simulink model "Approach2_ADAS_SimuEnv_Students"  (R2023b)
settings: Solver=FixedStepDiscrete  StartTime=0.0  StopTime=Time(end)  FixedStep=Te  RelTol=1e-3
undefined symbols (not defined in the file): b, DiscIntNeverNeededParam, phieq, phiini, Te, xini, yini
settings Model: Creator=a004139  LastModifiedBy=merte
settings SolverCC: AlgebraicLoopSolver=TrustRegion
settings DataIOCC: SaveOutput=off  SignalLogging=off  DSMLogging=off  SaveTime=off  ReturnWorkspaceOutputs=off  ReturnWorkspaceOutputsName=SimOut
settings DebuggingCC: UnconnectedInputMsg=warning  UnconnectedOutputMsg=warning  UnconnectedLineMsg=warning
settings ModelReferenceCC: EnableRefExpFcnMdlSchedulingChecks=on
settings RTWCC: DLArmComputeVersion=19.05

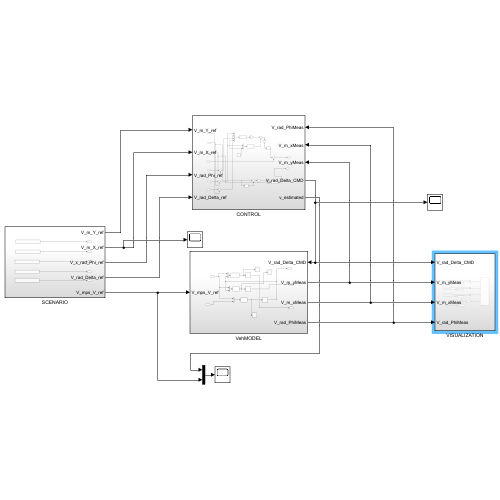
[thumbnail: Simulink's stored preview of the top-level diagram]
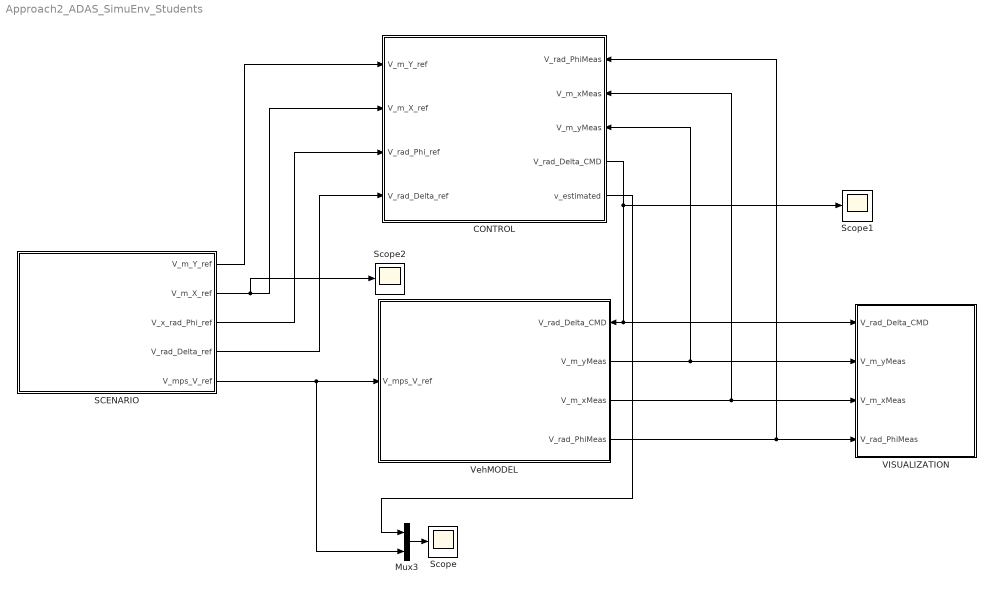
== system Approach2_ADAS_SimuEnv_Students ==
  CONTROL : Subsystem
      settings: PortSchema="{\"entries\":[{\"content\":{\"sides\":[{\"content\":{\"connectorIds\":[\"In1\",\"In2\",\"In3\",\"In4\"]},\"type\":\"ConnectorPlacement.EquallySpacedRectSide\",\"uuid\":\"0f23f3c4-7533-49c9-95fd-578963f4a754\"},{\"content\":{\"connectorIds\":[\"In5\",\"In6\",\"In7\",\"Out1\",\"Out2\"],\"side\":\"RIGHT\"},\"type\":\"ConnectorPlacement.EquallySpacedRectSide\",\"uuid\":\"9ec2fbe1-bc80-46e0-b9ca-3ad9a8a7d04a\"},{\"content\":{\"side\":\"TOP\"},\"type\":\"ConnectorPlacement.EquallySpacedRectSide\",\"uuid\":\"b91c010f-db5d-47ed-ad65-4a9135c33450\"}]},\"type\":\"ConnectorPlacement.EquallySpacedConnector\",\"uuid\":\"9aa72db9-4388-4ef7-aaa1-98aa5bf9b2fd\"}],\"packageUris\":[\"http://schema.mathworks.com/mf0/Connector/R2020b\"],\"version\":\"1.0\"}"
  Mux3 : Mux  Inputs=2
  SCENARIO : Subsystem
  Scope : Scope
  Scope1 : Scope
  Scope2 : Scope
  VISUALIZATION : Subsystem
  VehMODEL : Subsystem
      settings: PortSchema="{\"entries\":[{\"content\":{\"sides\":[{\"content\":{\"connectorIds\":[\"In1\"]},\"type\":\"ConnectorPlacement.EquallySpacedRectSide\",\"uuid\":\"e6ef4d01-9638-4fdb-8c0a-c1ee8e722df4\"},{\"content\":{\"connectorIds\":[\"In2\",\"Out1\",\"Out2\",\"Out3\"],\"side\":\"RIGHT\"},\"type\":\"ConnectorPlacement.EquallySpacedRectSide\",\"uuid\":\"6972533f-7f2e-4789-8f84-d3fb49c6524b\"},{\"content\":{\"connectorIds\":[],\"side\":\"TOP\"},\"type\":\"ConnectorPlacement.EquallySpacedRectSide\",\"uuid\":\"951c69a8-1198-4c47-a229-4417a6b3cd86\"}]},\"type\":\"ConnectorPlacement.EquallySpacedConnector\",\"uuid\":\"cfd1f762-b1bc-4353-bff3-d3c187fb9f94\"}],\"packageUris\":[\"http://schema.mathworks.com/mf0/Connector/19700101\"],\"version\":\"1.0\"}"
  wires:
  SCENARIO/5(V_mps_V_ref) -> VehMODEL/1(V_mps_V_ref), Mux3/2
  VehMODEL/1(V_m_yMeas) -> CONTROL/7(V_m_yMeas), VISUALIZATION/2(V_m_yMeas)
  VehMODEL/2(V_m_xMeas) -> CONTROL/6(V_m_xMeas), VISUALIZATION/3(V_m_xMeas)
  VehMODEL/3(V_rad_PhiMeas) -> CONTROL/5(V_rad_PhiMeas), VISUALIZATION/4(V_rad_PhiMeas)
  SCENARIO/1(V_m_Y_ref) -> CONTROL/1(V_m_Y_ref)
  SCENARIO/2(V_m_X_ref) -> Scope2/1, CONTROL/2(V_m_X_ref)
  SCENARIO/3(V_x_rad_Phi_ref) -> CONTROL/3(V_rad_Phi_ref)
  SCENARIO/4(V_rad_Delta_ref) -> CONTROL/4(V_rad_Delta_ref)
  CONTROL/1(V_rad_Delta_CMD) -> Scope1/1, VISUALIZATION/1(V_rad_Delta_CMD), VehMODEL/2(V_rad_Delta_CMD)
  Mux3/1 -> Scope/1
  CONTROL/2(v_estimated) -> Mux3/1

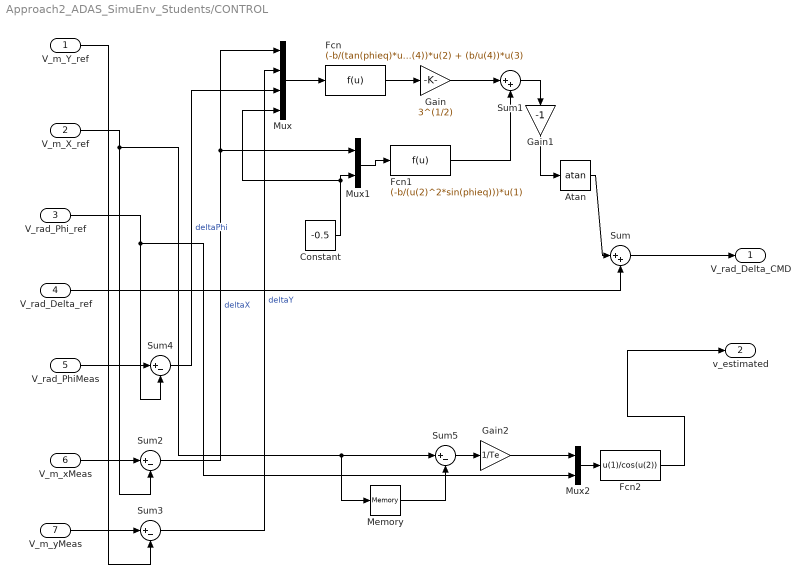
== system Approach2_ADAS_SimuEnv_Students/CONTROL ==
  V_m_Y_ref : Inport  PortDimensions=1
  V_m_X_ref : Inport  Port=2  PortDimensions=1
  V_rad_Phi_ref : Inport  Port=3  PortDimensions=1
  V_rad_Delta_ref : Inport  Port=4  PortDimensions=1
  V_rad_PhiMeas : Inport  Port=5  PortDimensions=1
  V_m_xMeas : Inport  Port=6  PortDimensions=1
  V_m_yMeas : Inport  Port=7  PortDimensions=1
  Atan : Trigonometry  Operator=atan
  Constant : Constant  Value=-0.5
  Fcn : Fcn  Expr=(-b/(tan(phieq)*u(4)))*u(1) + (-b/u(4))*u(2) + (b/u(4))*u(3)
  Fcn1 : Fcn  Expr=(-b/(u(2)^2*sin(phieq)))*u(1)
  Fcn2 : Fcn  Expr=u(1)/cos(u(2))
  Gain : Gain  Gain=3^(1/2)
  Gain1 : Gain  Gain=-1
  Gain2 : Gain  Gain=1/Te
  Memory : Memory  InitialCondition=0.0000001
  Mux : Mux
  Mux1 : Mux  Inputs=2
  Mux2 : Mux  Inputs=2
  Sum : Sum  Inputs=|++
  Sum1 : Sum  Inputs=|++
  Sum{2..5} (4 alike) : Sum  Inputs=|+-
  V_rad_Delta_CMD : Outport
  v_estimated : Outport  Port=2
  wires:
  Mux/1 -> Fcn/1
  Fcn/1 -> Gain/1
  Gain/1 -> Sum1/1
  V_m_xMeas/1 -> Sum2/1
  V_m_X_ref/1 -> Memory/1, Sum5/1, Sum2/2
  Sum2/1 -> Mux/1, Mux1/1  "deltaX"
  V_m_yMeas/1 -> Sum3/1
  V_m_Y_ref/1 -> Sum3/2
  Sum3/1 -> Mux/2  "deltaY"
  V_rad_PhiMeas/1 -> Sum4/1
  V_rad_Phi_ref/1 -> Mux2/2, Sum4/2
  Sum4/1 -> Mux/3  "deltaPhi"
  Mux1/1 -> Fcn1/1
  Fcn1/1 -> Sum1/2
  Sum1/1 -> Gain1/1
  Gain1/1 -> Atan/1
  Atan/1 -> Sum/1
  V_rad_Delta_ref/1 -> Sum/2
  Fcn2/1 -> v_estimated/1
  Memory/1 -> Sum5/2
  Gain2/1 -> Mux2/1
  Sum5/1 -> Gain2/1
  Mux2/1 -> Fcn2/1
  Sum/1 -> V_rad_Delta_CMD/1
  Constant/1 -> Mux/4, Mux1/2

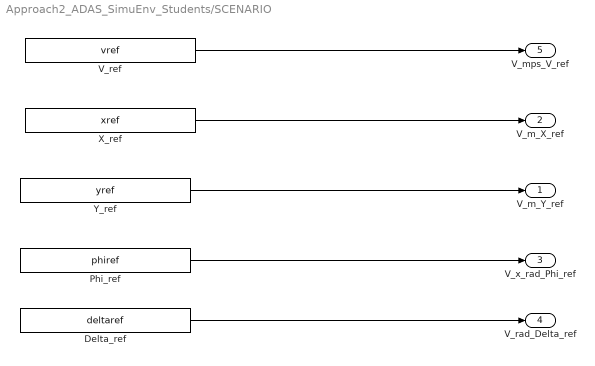
== system Approach2_ADAS_SimuEnv_Students/SCENARIO ==
  Delta_ref : FromWorkspace  VariableName=deltaref  SampleTime=Te  OutputAfterFinalValue=Holding final value
  Phi_ref : FromWorkspace  VariableName=phiref  SampleTime=Te  OutputAfterFinalValue=Holding final value
  V_ref : FromWorkspace  VariableName=vref  SampleTime=Te  OutputAfterFinalValue=Holding final value
  X_ref : FromWorkspace  VariableName=xref  SampleTime=Te  OutputAfterFinalValue=Holding final value
  Y_ref : FromWorkspace  VariableName=yref  SampleTime=Te  OutputAfterFinalValue=Holding final value
  V_m_Y_ref : Outport
  V_m_X_ref : Outport  Port=2
  V_x_rad_Phi_ref : Outport  Port=3
  V_rad_Delta_ref : Outport  Port=4
  V_mps_V_ref : Outport  Port=5
  wires:
  Phi_ref/1 -> V_x_rad_Phi_ref/1
  Y_ref/1 -> V_m_Y_ref/1
  V_ref/1 -> V_mps_V_ref/1
  Delta_ref/1 -> V_rad_Delta_ref/1
  X_ref/1 -> V_m_X_ref/1

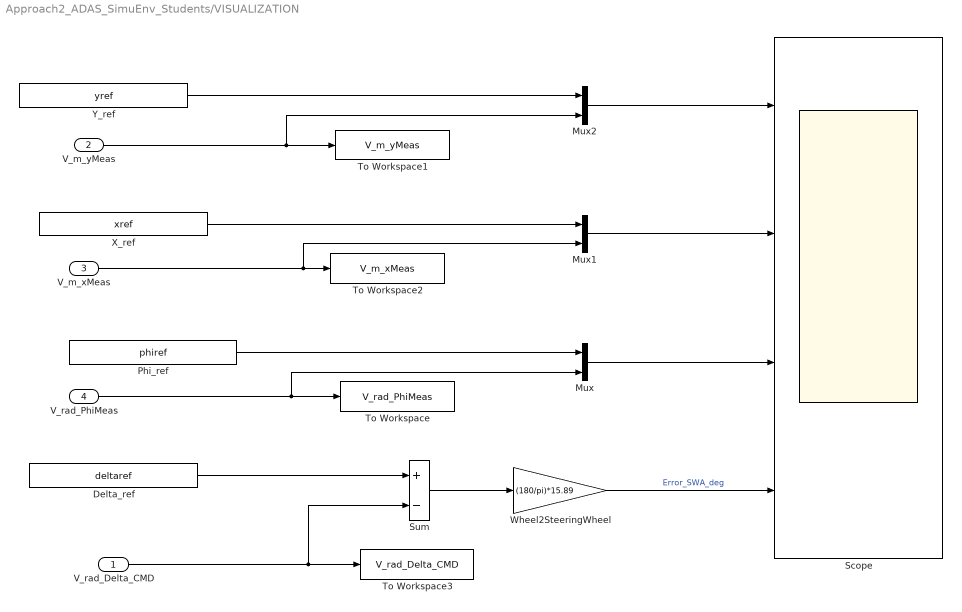
== system Approach2_ADAS_SimuEnv_Students/VISUALIZATION ==
  V_rad_Delta_CMD : Inport
  V_m_yMeas : Inport  Port=2
  V_m_xMeas : Inport  Port=3
  V_rad_PhiMeas : Inport  Port=4
  Delta_ref : FromWorkspace  VariableName=deltaref  SampleTime=Te  OutputAfterFinalValue=Holding final value
  Mux : Mux  Inputs=2
  Mux1 : Mux  Inputs=2
  Mux2 : Mux  Inputs=2
  Phi_ref : FromWorkspace  VariableName=phiref  SampleTime=Te  OutputAfterFinalValue=Holding final value
  Scope : Scope  NumInputPorts=4
  Sum : Sum  Inputs=+-
  To Workspace : ToWorkspace  VariableName=V_rad_PhiMeas  SaveFormat=Timeseries  SampleTime=Te
  To Workspace1 : ToWorkspace  VariableName=V_m_yMeas  SaveFormat=Timeseries  SampleTime=Te
  To Workspace2 : ToWorkspace  VariableName=V_m_xMeas  SaveFormat=Timeseries  SampleTime=Te
  To Workspace3 : ToWorkspace  VariableName=V_rad_Delta_CMD  SaveFormat=Timeseries  SampleTime=Te
  Wheel2SteeringWheel : Gain  Gain=(180/pi)*15.89
  X_ref : FromWorkspace  VariableName=xref  SampleTime=Te  OutputAfterFinalValue=Holding final value
  Y_ref : FromWorkspace  VariableName=yref  SampleTime=Te  OutputAfterFinalValue=Holding final value
  wires:
  V_rad_Delta_CMD/1 -> To Workspace3/1, Sum/2
  V_m_yMeas/1 -> Mux2/2, To Workspace1/1
  V_m_xMeas/1 -> Mux1/2, To Workspace2/1
  V_rad_PhiMeas/1 -> Mux/2, To Workspace/1
  Sum/1 -> Wheel2SteeringWheel/1
  Delta_ref/1 -> Sum/1
  Wheel2SteeringWheel/1 -> Scope/4  "Error_SWA_deg"
  Mux/1 -> Scope/3
  Mux1/1 -> Scope/2
  Mux2/1 -> Scope/1
  Y_ref/1 -> Mux2/1
  X_ref/1 -> Mux1/1
  Phi_ref/1 -> Mux/1

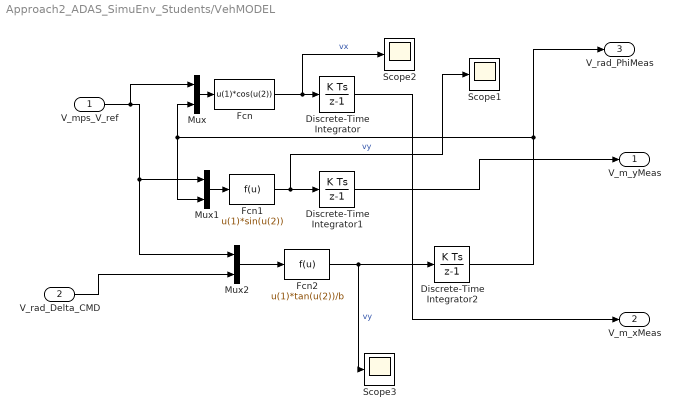
== system Approach2_ADAS_SimuEnv_Students/VehMODEL ==
  V_mps_V_ref : Inport  PortDimensions=1
  V_rad_Delta_CMD : Inport  Port=2  PortDimensions=1
  Discrete-Time Integrator : DiscreteIntegrator  InitialCondition=xini  SampleTime=Te  ICPrevOutput=DiscIntNeverNeededParam  ICPrevScaledInput=DiscIntNeverNeededParam
  Discrete-Time Integrator1 : DiscreteIntegrator  InitialCondition=yini  SampleTime=Te  ICPrevOutput=DiscIntNeverNeededParam  ICPrevScaledInput=DiscIntNeverNeededParam
  Discrete-Time Integrator2 : DiscreteIntegrator  InitialCondition=phiini  SampleTime=Te  ICPrevOutput=DiscIntNeverNeededParam  ICPrevScaledInput=DiscIntNeverNeededParam
  Fcn : Fcn  Expr=u(1)*cos(u(2))
  Fcn1 : Fcn  Expr=u(1)*sin(u(2))
  Fcn2 : Fcn  Expr=u(1)*tan(u(2))/b
  Mux : Mux  Inputs=2
  Mux1 : Mux  Inputs=2
  Mux2 : Mux  Inputs=2
  Scope1 : Scope
  Scope2 : Scope
  Scope3 : Scope
  V_m_yMeas : Outport
  V_m_xMeas : Outport  Port=2
  V_rad_PhiMeas : Outport  Port=3
  wires:
  V_mps_V_ref/1 -> Mux/1, Mux2/1, Mux1/1
  Fcn/1 -> Scope2/1, Discrete-Time Integrator/1  "vx"
  Fcn1/1 -> Scope1/1, Discrete-Time Integrator1/1  "vy"
  Discrete-Time Integrator/1 -> V_m_xMeas/1
  Discrete-Time Integrator1/1 -> V_m_yMeas/1
  Discrete-Time Integrator2/1 -> V_rad_PhiMeas/1, Mux1/2, Mux/2
  Mux/1 -> Fcn/1
  Mux1/1 -> Fcn1/1
  Fcn2/1 -> Scope3/1, Discrete-Time Integrator2/1  "vy"
  Mux2/1 -> Fcn2/1
  V_rad_Delta_CMD/1 -> Mux2/2
